simulink model "Linear_Controller"  (R2020a)
settings: Solver=VariableStepAuto  StartTime=0.0  StopTime=10.0  RelTol=1e-3
values from neighbouring files (symbols this model uses):
  F = [f1 , 0 ... (first row only)    [parameters.m]
  Kd = [10, 0 ... (first row only)    [parameters.m]
  Kp = [30 , 0 ... (first row only)    [parameters.m]
settings Model: Creator=sirius  LastModifiedBy=sirius

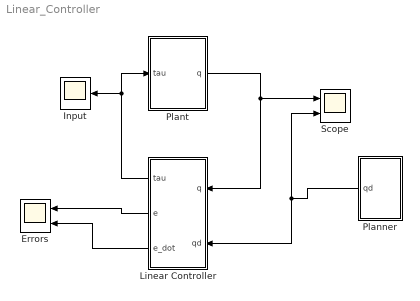
== system Linear_Controller ==
  Errors : Scope  NumInputPorts=2
  Input : Scope
  Linear Controller : Subsystem
  Planner : Subsystem
  Plant : Subsystem
  Scope : Scope  NumInputPorts=2
  wires:
  Plant/1(q) -> Linear Controller/1(q), Scope/1
  Planner/1(qd) -> Scope/2, Linear Controller/2(qd)
  Linear Controller/1(tau) -> Plant/1(tau), Input/1
  Linear Controller/2(e) -> Errors/1
  Linear Controller/3(e_dot) -> Errors/2

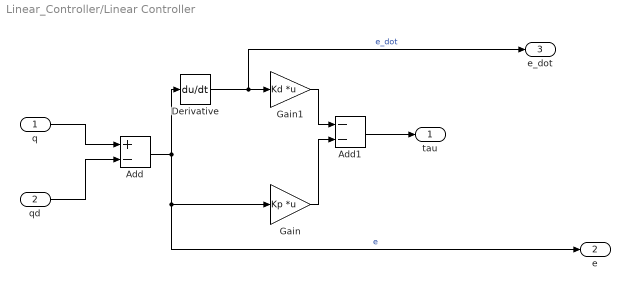
== system Linear_Controller/Linear Controller ==
  q : Inport
  qd : Inport  Port=2
  Add : Sum  Inputs=+-
  Add1 : Sum  Inputs=--
  Derivative : Derivative
  Gain : Gain  Gain=Kp  Multiplication=Matrix(K*u)
  Gain1 : Gain  Gain=Kd  Multiplication=Matrix(K*u)
  tau : Outport
  e : Outport  Port=2
  e_dot : Outport  Port=3
  wires:
  q/1 -> Add/1
  qd/1 -> Add/2
  Add/1 -> e/1, Gain/1, Derivative/1  "e"
  Derivative/1 -> e_dot/1, Gain1/1  "e_dot"
  Gain1/1 -> Add1/1
  Gain/1 -> Add1/2
  Add1/1 -> tau/1

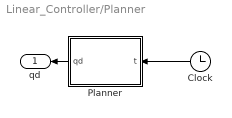
== system Linear_Controller/Planner ==
  Clock : Clock
  Planner : MATLAB Function  TreatAsAtomicUnit=on
  qd : Outport
  wires:
  Clock/1 -> Planner/1(t)
  Planner/1(qd) -> qd/1

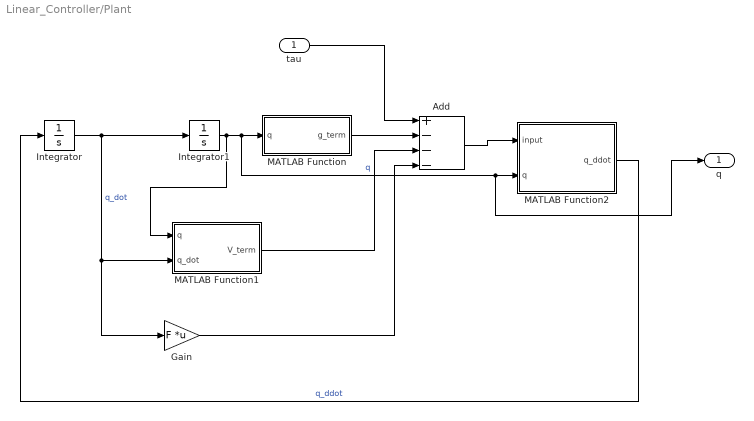
== system Linear_Controller/Plant ==
  tau : Inport
  Add : Sum  Inputs=+---
  Gain : Gain  Gain=F  Multiplication=Matrix(K*u)
  Integrator : Integrator
  Integrator1 : Integrator  InitialCondition=[0;0]
  MATLAB Function : MATLAB Function  TreatAsAtomicUnit=on
  MATLAB Function1 : MATLAB Function  TreatAsAtomicUnit=on
  MATLAB Function2 : MATLAB Function  TreatAsAtomicUnit=on
  q : Outport
  wires:
  MATLAB Function2/1(q_ddot) -> Integrator/1  "q_ddot"
  MATLAB Function/1(g_term) -> Add/2
  Add/1 -> MATLAB Function2/1(input)
  MATLAB Function1/1(V_term) -> Add/3
  Integrator/1 -> Gain/1, MATLAB Function1/2(q_dot), Integrator1/1  "q_dot"
  tau/1 -> Add/1
  Gain/1 -> Add/4
  Integrator1/1 -> MATLAB Function1/1(q), q/1, MATLAB Function2/2(q), MATLAB Function/1(q)  "q"

== matlab function Linear_Controller/Plant/MATLAB Function ==
  data: q input; g_term output
function g_term = G(q)
g_term = [35.9929*cos(q(1)) + 1.92276*cos(q(1) + q(2));
          1.92276*cos(q(1) + q(2));];

== matlab function Linear_Controller/Plant/MATLAB Function2 ==
  data: input input; q_ddot output; q input
function q_ddot = M_inverse(input,q)
M = [ (49*cos(q(2)))/125 + 773/200, (49*cos(q(2)))/250 + 49/250;
   (49*cos(q(2)))/250 + 49/250,                    49/250;];
q_ddot = M\input;
end

== matlab function Linear_Controller/Planner/Planner ==
  data: t input; qd output
function qd = Traj(t)
qd = [pi/3 + pi/6*sin(t);
      pi/4 + pi/6*cos(t)];

== matlab function Linear_Controller/Plant/MATLAB Function1 ==
  data: q input; V_term output; q_dot input
function V_term = V(q,q_dot)

V_term = [-0.196*(2*q_dot(1)*q_dot(2) + q_dot(2)^2)*sin(q(2));
            0.196*q_dot(1)^2*sin(q(2))];
end
